simulink model "soler_sytem_only_with_inverter"  (R2020a)
settings: Solver=VariableStepAuto  StartTime=0.0  StopTime=.05  RelTol=1e-3
libraries: powerlib x15, re_lib x1
settings Model: Creator=hp  LastModifiedBy=hp

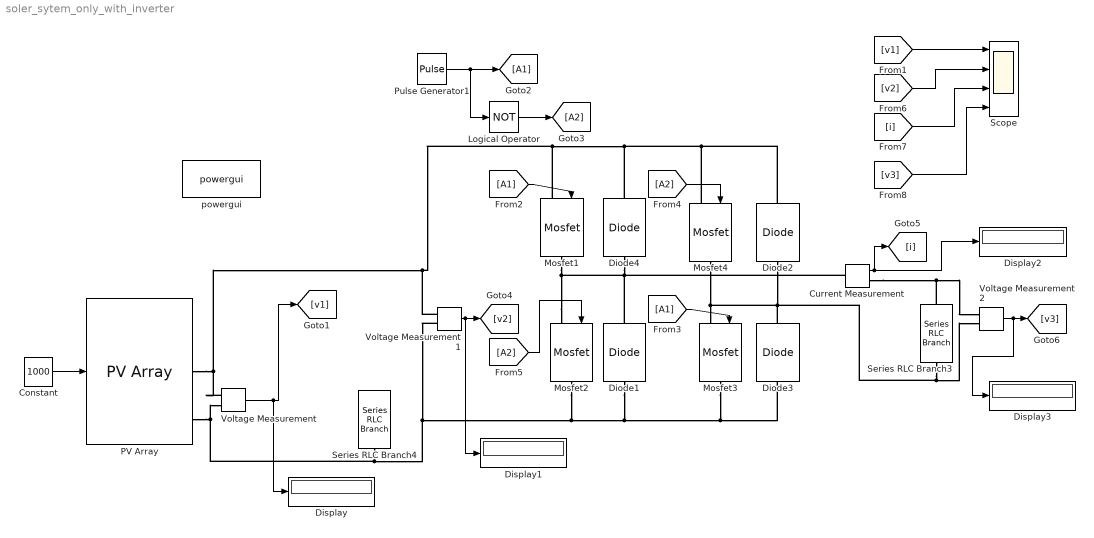
== system soler_sytem_only_with_inverter ==
  Constant : Constant  Value=1000
  Current Measurement : powerlib/Measurements/Current Measurement  PhasorSimulation=off  OutputType=Complex  PSBequivalent=0
  Diode{1..4} (4 alike) : powerlib/Power Electronics/Diode  Ron=0.001  Lon=0  Vf=0.8  IC=0  UseSnubber=0  Rs=500  Cs=250e-9  Measurements=off
  Display{,1..3} (4 alike) : Display
  Logical Operator : Logic  Operator=NOT  AllPortsSameDT=off  OutDataTypeStr=boolean
  Mosfet{1..4} (4 alike) : powerlib/Power Electronics/Mosfet  Ron=0.1  Lon=0  Rd=0.01  Vfd=0  IC=0  Rs=1e5  Cs=inf  Measurements=off
  PV Array : re_lib/Solar/PV Array  Npar=1  Nser=10  PlotType=array @ 1000 W/m2 & specified temperatures  S_vec="[ 1000  500  100 ]"  Temp_C_vec="[ 45 25  ]"  ModuleName=1Soltech 1STH-215-P  PlotWhenSelected=off  Pm=213.15  Ncell=60  Voc=36.3  Isc=7.84  Vm=29  Im=7.35  beta_Voc_pc=-0.36099  alpha_Isc_pc=0.102  beta_Voc=-0.13104  alpha_Isc=0.007997  IL=7.8649  I0=2.9259e-10  nI=0.98117  Rsh=313.3991  Rs=0.39383  RobustModel=on  RobustCellTemperature=25  BAL=on  Tc=1e-6  Tfilter=5e-5
  Pulse Generator1 : DiscretePulseGenerator  PulseType=Time based  Period=1/50  PulseWidth=50
  Scope : Scope  NumInputPorts=4
  Series RLC Branch3 : powerlib/Elements/Series RLC Branch  LConnTagsString=__new0  RConnTagsString=__new0  BranchType=R  Resistance=45  Inductance=1e-3  SetiL0=off  InitialCurrent=0  Capacitance=1e-6  Setx0=off  InitialVoltage=0  Measurements=None
  Series RLC Branch4 : powerlib/Elements/Series RLC Branch  LConnTagsString=__new0  RConnTagsString=__new0  BranchType=C  Resistance=1  Inductance=1e-3  SetiL0=off  InitialCurrent=0  Capacitance=.050689655  Setx0=off  InitialVoltage=0  Measurements=None
  Voltage Measurement : powerlib/Measurements/Voltage Measurement  PhasorSimulation=off  OutputType=Complex  PSBequivalent=0
  Voltage Measurement1 : powerlib/Measurements/Voltage Measurement  PhasorSimulation=off  OutputType=Complex  PSBequivalent=0
  Voltage Measurement2 : powerlib/Measurements/Voltage Measurement  PhasorSimulation=off  OutputType=Complex  PSBequivalent=0
  powergui : powerlib/powergui  Priority=1  SimulationMode=Discrete  SampleTime=50e-6  frequency=60  Iterations=50  frequencyindice=0  Pbase=100e6  ErrMax=1e-4  UnitsV=kV  UnitsW=MW  buscounter=0  FunctionMessages=off  echomessages=off  EnableUseOfTLC=off  CurrentSourceSwitches=off  DisableSnubberDevices=off  DisableRonSwitches=off  DisableVfSwitches=off  DisplayEquations=off  AutomaticDiscreteSolvers=off  SolverType=Tustin/Backward Euler (TBE)  Interpol=off  ExternalGateDelay=off  methode=off  Ts=100  x0status=blocks  SPID=on  SwTol=0  HookPort=off  NonlinearTolerance=1e-4  nMaxIteration=100  ContinueOnMaxIteration=off  RestoreLinks=warning  ResistiveCurrentMeasurement=off  Frange=[0:2:500]  Ylog=off  Xlog=on  ShowGrid=off  save=off  variable=ZData  structure=0  ZoomFFT=off  StartTime=0.0  cycles=1  DisplayStyle=1  fundamental=60  FreqAxis=off  MaxFrequency=1000  frequencyindicesteady=1  RmsSteady=1  display=off
  wires:
  [A1] -> Mosfet1/1
  [i] -> Scope/3
  [v2] -> Scope/2
  [v3] -> Scope/4
  Pulse Generator1/1 -> [A1], Logical Operator/1
  Logical Operator/1 -> [A2]
  [A2] -> Mosfet2/1
  [A1] -> Mosfet3/1
  Voltage Measurement1/1 -> Display1/1, [v2]
  Current Measurement/1 -> [i], Display2/1
  [A2] -> Mosfet4/1
  [v1] -> Scope/1
  Voltage Measurement2/1 -> Display3/1, [v3]
  Constant/1 -> PV Array/1
  Voltage Measurement/1 -> [v1], Display/1
  connections:
  PV Array/RConn2 -- Series RLC Branch4/RConn1 -- Voltage Measurement1/LConn2 -- Diode1/LConn1 -- Mosfet3/RConn1 -- Diode3/LConn1 -- Mosfet2/RConn1 -- Voltage Measurement/LConn2
  Series RLC Branch3/LConn1 -- Current Measurement/RConn1 -- Voltage Measurement2/LConn1
  Voltage Measurement/LConn1 -- Voltage Measurement1/LConn1 -- Mosfet4/LConn1 -- Diode2/RConn1 -- Diode4/RConn1 -- Mosfet1/LConn1 -- PV Array/RConn1
  Mosfet2/LConn1 -- Current Measurement/LConn1 -- Diode4/LConn1 -- Diode1/RConn1 -- Mosfet1/RConn1
  Series RLC Branch3/RConn1 -- Diode3/RConn1 -- Diode2/LConn1 -- Mosfet4/RConn1 -- Mosfet3/LConn1 -- Voltage Measurement2/LConn2
